simulink model "stateflowLearning"  (R2020b)
settings: Solver=VariableStepAuto  StartTime=0.0  StopTime=10.0  RelTol=1e-3
settings Model: Creator=masdoua1  LastModifiedBy=masdoua1

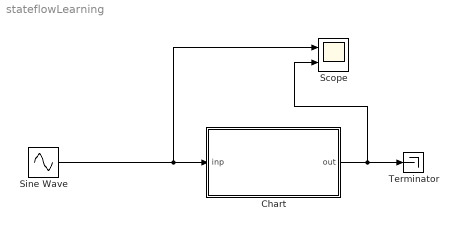
== system stateflowLearning ==
  Chart : Stateflow chart  TreatAsAtomicUnit=on
  Scope : Scope  NumInputPorts=2
  Sine Wave : Sin  SampleTime=0
  Terminator : Terminator
  wires:
  Sine Wave/1 -> Scope/1, Chart/1(inp)
  Chart/1(out) -> Scope/2, Terminator/1

== stateflow chart stateflowLearning/Chart ==
  state Off
    entry:
    out = 1;% action1
  state On
    entry:
    out=2; %action 2
  (default) -> Off
  Off -> On : [inp >0]
      | %transition 1
  On -> Off : [inp <=0]
      | %transition2
  data: inp input; out output
